simulink model "ControlTorque"  (R2013a)
settings: Solver=FixedStepDiscrete  StartTime=0.0  StopTime=inf  FixedStep=robot.Ts  RelTol=1e-3
values from neighbouring files (symbols this model uses):
  control = struct    [init.m]
  Reference = struct    [init.m]
  robot = robot.loadData('ref')    [init.m]
undefined symbols (not defined in the file or in its folder): motor, ROBOT_DOF
libraries: WBCLibrary x20, dspmtrx3 x2, simulink x1
settings Model: Creator=Raffaello  LastModifiedBy=Raffaello
settings DebuggingCC: InheritedTsInSrcMsg=none

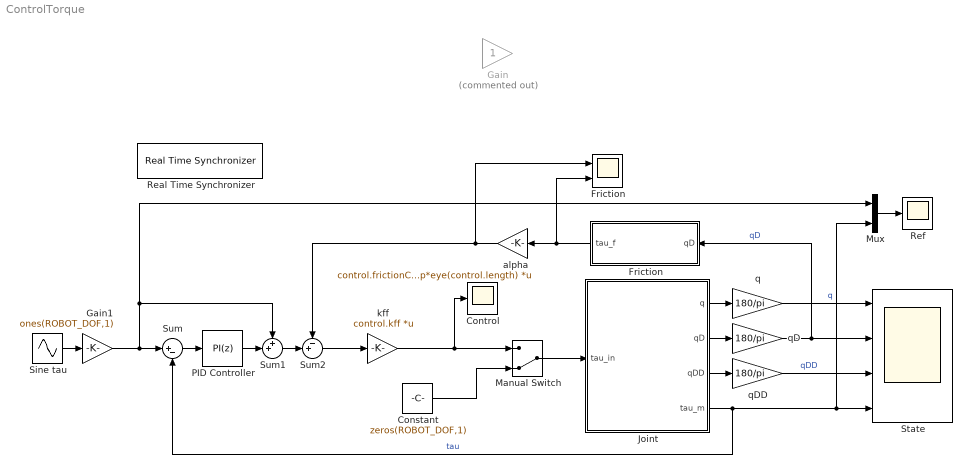
== system ControlTorque ==
  Constant : Constant  Value=zeros(ROBOT_DOF,1)
  Control : Scope
      settings: TimeRange=120  YMin=-44  YMax=-24  SaveName=ScopeData6
  Friction : Scope  NumInputPorts=2
      settings: TimeRange=120  YMin=-1~-5  YMax=2.25~5  SaveName=ScopeData7
  "Friction " : Subsystem
  Gain : Gain  Commented=on
  Gain1 : Gain  Gain=ones(ROBOT_DOF,1)
  Joint : Subsystem
  Manual Switch : ManualSwitch  CurrentSetting=0
  Mux : Mux  Inputs=2
  PID Controller : simulink/Continuous/PID Controller  Controller=PI  TimeDomain=Discrete-time  SampleTime=robot.Ts  IntegratorMethod=Trapezoidal  FilterMethod=Forward Euler  Form=Parallel  P=1  I=0  D=0  N=100  InitialConditionSource=internal  InitialConditionForIntegrator=0  InitialConditionForFilter=0  ExternalReset=none  LimitOutput=off  UpperSaturationLimit=inf  LowerSaturationLimit=-inf  LinearizeAsGain=on  AntiWindupMode=none  Kb=1  TrackingMode=off  Kt=1  PParamMin=[]  PParamMax=[]  IParamMin=[]  IParamMax=[]  DParamMin=[]  DParamMax=[]  NParamMin=[]  NParamMax=[]  KbParamMin=[]  KbParamMax=[]  KtParamMin=[]  KtParamMax=[]  POutMin=[]  POutMax=[]  IOutMin=[]  IOutMax=[]  DOutMin=[]  DOutMax=[]  NOutMin=[]  NOutMax=[]  KbOutMin=[]  KbOutMax=[]  KtOutMin=[]  KtOutMax=[]  IntegratorOutMin=[]  IntegratorOutMax=[]  FilterOutMin=[]  FilterOutMax=[]  SumOutMin=[]  SumOutMax=[]  SumI1OutMin=[]  SumI1OutMax=[]  SumI2OutMin=[]  SumI2OutMax=[]  SumI3OutMin=[]  SumI3OutMax=[]  SumDOutMin=[]  SumDOutMax=[]  SaturationOutMin=[]  SaturationOutMax=[]  IntegratorContinuousStateAttributes=''  IntegratorStateMustResolveToSignalObject=off  IntegratorRTWStateStorageClass=Auto  FilterContinuousStateAttributes=''  FilterStateMustResolveToSignalObject=off  FilterRTWStateStorageClass=Auto
  Real Time Synchronizer : WBCLibrary/Utilities/Real Time Synchronizer  Priority=-10  threadPeriod=robot.Ts
  Ref : Scope
      settings: TimeRange=120  YMin=-6  YMax=8  SaveName=ScopeData3
  Sine tau : Sin  Amplitude=Reference.sinAmp  Bias=Reference.sinBias  Frequency=Reference.sinFreq*2*pi  SampleTime=0
  State : Scope  NumInputPorts=4
      settings: ShowLegends=on  TimeRange=60  YMin=9.98~-0.3~-3~1.719  YMax=10.07~0.25~3.5~1.731  SaveName=ScopeData2
  Sum : Sum  Inputs=|+-
  Sum1 : Sum  Inputs=++|
  Sum2 : Sum  Inputs=-+|
  alpha : Gain  Gain=control.frictionComp*eye(control.length)  Multiplication=Matrix(K*u) (u vector)
  kff : Gain  Gain=control.kff  Multiplication=Matrix(K*u) (u vector)
  q : Gain  Gain=180/pi
  qD : Gain  Gain=180/pi
  qDD : Gain  Gain=180/pi
  wires:
  qD/1 -> "Friction "/1(qD), State/2  "qD"
  Mux/1 -> Ref/1
  q/1 -> State/1  "q"
  qDD/1 -> State/3  "qDD"
  Joint/4(tau_m) -> Sum/2, Mux/2, State/4  "tau"
  Joint/1(q) -> q/1
  Joint/2(qD) -> qD/1
  Joint/3(qDD) -> qDD/1
  Sine tau/1 -> Gain1/1
  Sum/1 -> PID Controller/1
  Sum1/1 -> Sum2/2
  Sum2/1 -> kff/1
  alpha/1 -> Sum2/1, Friction/1
  "Friction "/1(tau_f) -> alpha/1, Friction/2
  PID Controller/1 -> Sum1/2
  kff/1 -> Manual Switch/1, Control/1
  Constant/1 -> Manual Switch/2
  Gain1/1 -> Sum1/1, Mux/1, Sum/1
  Manual Switch/1 -> Joint/1(tau_in)

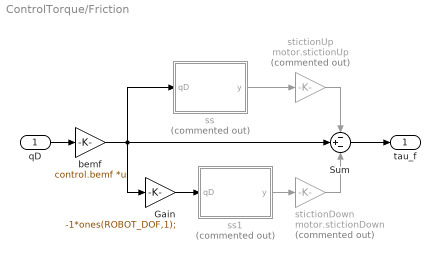
== system ControlTorque/Friction  ==
  qD : Inport
  Gain : Gain  Gain=-1*ones(ROBOT_DOF,1);
  Sum : Sum  Inputs=-+-
  bemf : Gain  Gain=control.bemf  Multiplication=Matrix(K*u) (u vector)
  ss : MATLAB Function  Commented=on  TreatAsAtomicUnit=on
  ss1 : MATLAB Function  Commented=on  TreatAsAtomicUnit=on
  stictionDown : Gain  Commented=on  Gain=motor.stictionDown
  stictionUp : Gain  Commented=on  Gain=motor.stictionUp
  tau_f : Outport
  wires:
  qD/1 -> bemf/1
  Sum/1 -> tau_f/1
  bemf/1 -> Gain/1, Sum/2, ss/1(qD)
  ss/1(y) -> stictionUp/1
  stictionUp/1 -> Sum/1
  ss1/1(y) -> stictionDown/1
  stictionDown/1 -> Sum/3
  Gain/1 -> ss1/1(qD)

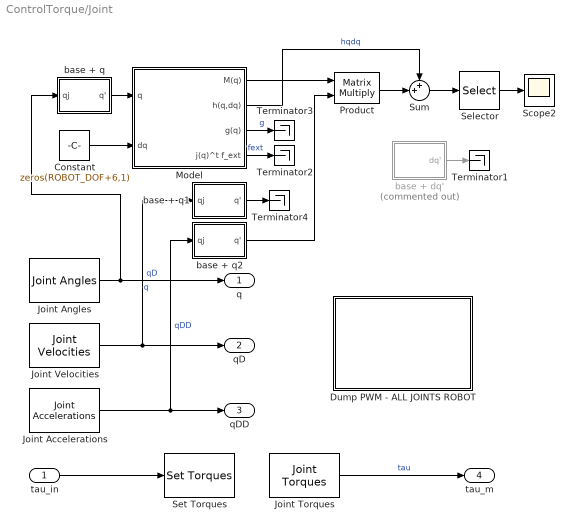
== system ControlTorque/Joint ==
  tau_in : Inport
  Constant : Constant  Value=zeros(ROBOT_DOF+6,1)
  Dump PWM - ALL JOINTS ROBOT : Subsystem  mask{output='getOutputs'}
      mask prompts: output "Output port"
      mask Display:
      | color('red'); plot([10 20 30 40], [10 20 10 15]);
      | color('blue'); plot([10 20 30 40], [15 10 20 12]);
      | color('green'); plot([10 20 30 40], [13 16 12 18]);
  Joint Accelerations : WBCLibrary/wholeBodyStates/Joint Accelerations  robotName=robot.robotName  localName=robot.localName
  Joint Angles : WBCLibrary/wholeBodyStates/Joint Angles  robotName=robot.robotName  localName=robot.localName
  Joint Torques : WBCLibrary/wholeBodyStates/Joint Torques  robotName=robot.robotName  localName=robot.localName
  Joint Velocities : WBCLibrary/wholeBodyStates/Joint Velocities  robotName=robot.robotName  localName=robot.localName
  Model : Subsystem
  Product : Product  Multiplication=Matrix(*)
  Scope2 : Scope
      settings: YMin=-50  YMax=300  SaveName=ScopeData4
  Selector : Selector  InputPortWidth=ROBOT_DOF+6  IndexOptions=Index vector (dialog)  Indices=[7]  OutputSizes=1
  Set Torques : WBCLibrary/wholeBodyActuators/Set Torques  val=6  robotName=robot.robotName  localName=robot.localName
  Sum : Sum  Inputs=++|
  Terminator{1..4} (4 alike) : Terminator
  base + dq' : Subsystem  Commented=on
  base + q : Subsystem
  base + q1 : Subsystem
  base + q2 : Subsystem
  q : Outport
  qD : Outport  Port=2
  qDD : Outport  Port=3
  tau_m : Outport  Port=4
  wires:
  Model/1(M(q)) -> Product/1
  Joint Accelerations/1 -> qDD/1, base + q2/1(qj)  "qDD"
  Joint Velocities/1 -> qD/1, base + q1/1(qj)  "qD"
  Constant/1 -> Model/2(dq)
  Joint Angles/1 -> q/1, base + q/1(qj)  "q"
  base + q1/1(q') -> Terminator4/1
  Selector/1 -> Scope2/1
  Model/4(j(q)^t f_ext) -> Terminator2/1  "fext"
  base + q/1(q') -> Model/1(q)
  Model/3(g(q)) -> Terminator3/1  "g"
  Joint Torques/1 -> tau_m/1  "tau"
  Sum/1 -> Selector/1
  Model/2(h(q,dq)) -> Sum/1  "hqdq"
  Product/1 -> Sum/2
  tau_in/1 -> Set Torques/1
  base + dq'/1(dq') -> Terminator1/1
  base + q2/1(q') -> Product/2

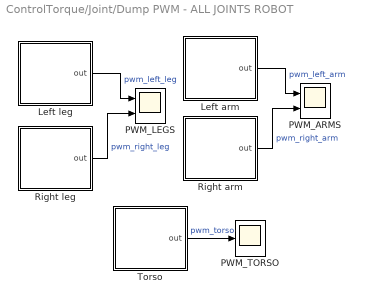
== system ControlTorque/Joint/Dump PWM - ALL JOINTS ROBOT ==
  Left arm : Subsystem  mask{type_arm='left_arm', output=output}
      mask prompts: type_arm "Type leg"; output "Output Port"
  Left leg : Subsystem  mask{type_arm='left_leg', output=output}
      mask prompts: type_arm "Type leg"; output "Output port"
  PWM_ARMS : Scope  NumInputPorts=2
      settings: TimeRange=60  YMin=-10~-10  YMax=12.5~15
  PWM_LEGS : Scope  NumInputPorts=2
      settings: TimeRange=60  YMin=-10~-10  YMax=12.5~15
  PWM_TORSO : Scope
      settings: TimeRange=60  YMin=-10  YMax=12.5  SaveName=ScopeData5
  Right arm : Subsystem  mask{type_arm='right_arm', output=output}
      mask prompts: type_arm "Type leg"; output "Output Port"
  Right leg : Subsystem  mask{type_arm='right_leg', output=output}
      mask prompts: type_arm "Type leg"; output "Output port"
  Torso : Subsystem  mask{type_arm='torso', output=output}
      mask prompts: type_arm "Type leg"; output "Output port"
  wires:
  Left arm/1(out) -> PWM_ARMS/1  "pwm_left_arm"
  Right arm/1(out) -> PWM_ARMS/2  "pwm_right_arm"
  Torso/1(out) -> PWM_TORSO/1  "pwm_torso"
  Right leg/1(out) -> PWM_LEGS/2  "pwm_right_leg"
  Left leg/1(out) -> PWM_LEGS/1  "pwm_left_leg"

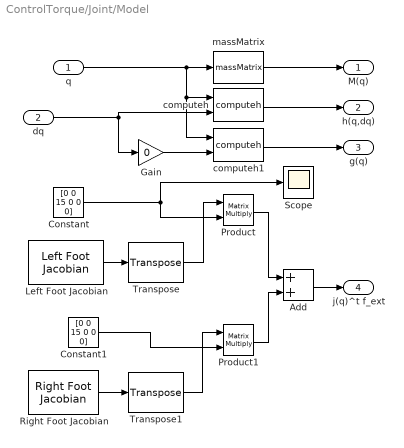
== system ControlTorque/Joint/Model ==
  q : Inport
  dq : Inport  Port=2
  Add : Sum
  Constant : Constant  Value=[0 0 15 0 0 0]
  Constant1 : Constant  Value=[0 0 15 0 0 0]
  Gain : Gain  Gain=0
  Left Foot Jacobian : WBCLibrary/wholeBodyModel/Jacobians/Left Foot Jacobian  robotName=robot.robotName  localName=robot.localName
  Product : Product  Multiplication=Matrix(*)
  Product1 : Product  Multiplication=Matrix(*)
  Right Foot Jacobian : WBCLibrary/wholeBodyModel/Jacobians/Right Foot Jacobian  robotName=robot.robotName  localName=robot.localName
  Scope : Scope
  Transpose : dspmtrx3/Transpose  Hermitian=off  overflowFlag=off
  Transpose1 : dspmtrx3/Transpose  Hermitian=off  overflowFlag=off
  computeh : WBCLibrary/wholeBodyModel/Dynamics/computeh  val=7  robotname=robot.robotName  localname=robot.localName
  computeh1 : WBCLibrary/wholeBodyModel/Dynamics/computeh  val=7  robotname=robot.robotName  localname=robot.localName
  massMatrix : WBCLibrary/wholeBodyModel/Dynamics/massMatrix  val=8  robotname=robot.robotName  localname=robot.localName
  M(q) : Outport
  h(q,dq) : Outport  Port=2
  g(q) : Outport  Port=3
  j(q)^t f_ext : Outport  Port=4
  wires:
  Gain/1 -> computeh1/2
  computeh1/1 -> g(q)/1
  computeh/1 -> h(q,dq)/1
  massMatrix/1 -> M(q)/1
  q/1 -> computeh1/1, computeh/1, massMatrix/1
  dq/1 -> computeh/2, Gain/1
  Left Foot Jacobian/1 -> Transpose/1
  Right Foot Jacobian/1 -> Transpose1/1
  Constant/1 -> Product/2, Scope/1
  Transpose/1 -> Product/1
  Constant1/1 -> Product1/2
  Transpose1/1 -> Product1/1
  Product/1 -> Add/1
  Product1/1 -> Add/2
  Add/1 -> j(q)^t f_ext/1

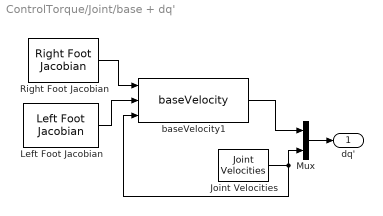
== system ControlTorque/Joint/base + dq' ==
  Joint Velocities : WBCLibrary/wholeBodyStates/Joint Velocities  robotName=robot.robotName  localName=robot.localName
  Left Foot Jacobian : WBCLibrary/wholeBodyModel/Jacobians/Left Foot Jacobian  robotName=robot.robotName  localName=robot.localName
  Mux : Mux  Inputs=2
  Right Foot Jacobian : WBCLibrary/wholeBodyModel/Jacobians/Right Foot Jacobian  robotName=robot.robotName  localName=robot.localName
  baseVelocity1 : WBCLibrary/Utilities/baseVelocity
  dq' : Outport
  wires:
  Left Foot Jacobian/1 -> baseVelocity1/2
  Right Foot Jacobian/1 -> baseVelocity1/1
  baseVelocity1/1 -> Mux/1
  Joint Velocities/1 -> baseVelocity1/3, Mux/2
  Mux/1 -> dq'/1

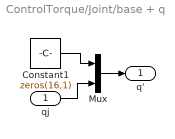
== system ControlTorque/Joint/base + q ==
  qj : Inport
  Constant1 : Constant  Value=zeros(16,1)
  Mux : Mux  Inputs=2
  q' : Outport
  wires:
  Mux/1 -> q'/1
  qj/1 -> Mux/2
  Constant1/1 -> Mux/1

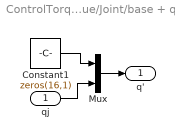
== system ControlTorque/Joint/base + q1 ==
  qj : Inport
  Constant1 : Constant  Value=zeros(16,1)
  Mux : Mux  Inputs=2
  q' : Outport
  wires:
  Mux/1 -> q'/1
  qj/1 -> Mux/2
  Constant1/1 -> Mux/1

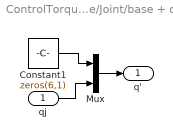
== system ControlTorque/Joint/base + q2 ==
  qj : Inport
  Constant1 : Constant  Value=zeros(6,1)
  Mux : Mux  Inputs=2
  q' : Outport
  wires:
  Constant1/1 -> Mux/1
  qj/1 -> Mux/2
  Mux/1 -> q'/1

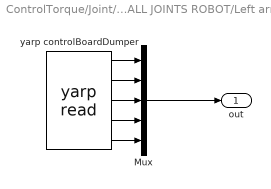
== system ControlTorque/Joint/Dump PWM - ALL JOINTS ROBOT/Left arm ==
  Mux : Mux  Inputs=5
  yarp controlBoardDumper : WBCLibrary/Utilities/yarp read  from=['/controlBoardDumper/' type_arm '/' output]  to='...'  num=5  blocking=off  timestamp=off
  out : Outport
  wires:
  Mux/1 -> out/1
  yarp controlBoardDumper/1 -> Mux/1
  yarp controlBoardDumper/3 -> Mux/3
  yarp controlBoardDumper/2 -> Mux/2
  yarp controlBoardDumper/5 -> Mux/5
  yarp controlBoardDumper/4 -> Mux/4

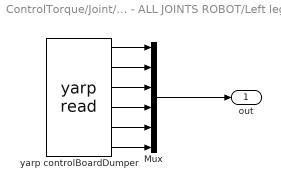
== system ControlTorque/Joint/Dump PWM - ALL JOINTS ROBOT/Left leg ==
  Mux : Mux  Inputs=6
  yarp controlBoardDumper : WBCLibrary/Utilities/yarp read  from=['/controlBoardDumper/' type_arm '/' output]  to='...'  num=6  blocking=off  timestamp=off
  out : Outport
  wires:
  Mux/1 -> out/1
  yarp controlBoardDumper/1 -> Mux/1
  yarp controlBoardDumper/3 -> Mux/3
  yarp controlBoardDumper/2 -> Mux/2
  yarp controlBoardDumper/5 -> Mux/5
  yarp controlBoardDumper/6 -> Mux/6
  yarp controlBoardDumper/4 -> Mux/4

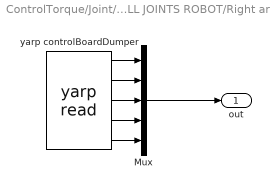
== system ControlTorque/Joint/Dump PWM - ALL JOINTS ROBOT/Right arm ==
  Mux : Mux  Inputs=5
  yarp controlBoardDumper : WBCLibrary/Utilities/yarp read  from=['/controlBoardDumper/' type_arm '/' output]  to='...'  num=5  blocking=off  timestamp=off
  out : Outport
  wires:
  Mux/1 -> out/1
  yarp controlBoardDumper/1 -> Mux/1
  yarp controlBoardDumper/3 -> Mux/3
  yarp controlBoardDumper/2 -> Mux/2
  yarp controlBoardDumper/5 -> Mux/5
  yarp controlBoardDumper/4 -> Mux/4

== system ControlTorque/Joint/Dump PWM - ALL JOINTS ROBOT/Right leg ==
  Mux : Mux  Inputs=6
  yarp controlBoardDumper : WBCLibrary/Utilities/yarp read  from=['/controlBoardDumper/' type_arm '/' output]  to='...'  num=6  blocking=off  timestamp=off
  out : Outport
  wires:
  Mux/1 -> out/1
  yarp controlBoardDumper/1 -> Mux/1
  yarp controlBoardDumper/3 -> Mux/3
  yarp controlBoardDumper/2 -> Mux/2
  yarp controlBoardDumper/5 -> Mux/5
  yarp controlBoardDumper/6 -> Mux/6
  yarp controlBoardDumper/4 -> Mux/4

== system ControlTorque/Joint/Dump PWM - ALL JOINTS ROBOT/Torso ==
  Mux : Mux  Inputs=3
  yarp controlBoardDumper : WBCLibrary/Utilities/yarp read  from=['/controlBoardDumper/' type_arm '/' output]  to='...'  num=3  blocking=off  timestamp=off
  out : Outport
  wires:
  Mux/1 -> out/1
  yarp controlBoardDumper/1 -> Mux/1
  yarp controlBoardDumper/3 -> Mux/3
  yarp controlBoardDumper/2 -> Mux/2

== matlab function ControlTorque/Friction /ss1 ==
  data: qD input; y output; qDth parameter
function y = ss(qD, qDth)
%#codegen

if qD < 0
   y = 0;
elseif qD > qDth
    y = 1;
else
    y = (qD/qDth)^3;
end

== matlab function ControlTorque/Friction /ss ==
  data: qD input; y output; qDth parameter
function y = ss(qD, qDth)
%#codegen

if qD < 0
   y = 0;
elseif qD > qDth
    y = 1;
else
    y = (qD/qDth)^3;
end
